simulink model "P3"  (Simulink 7.6)
settings: Solver=ode45  StartTime=0.0  StopTime=10.0  RelTol=1e-3
settings Model: Creator=USUARIO  LastModifiedBy=USUARIO

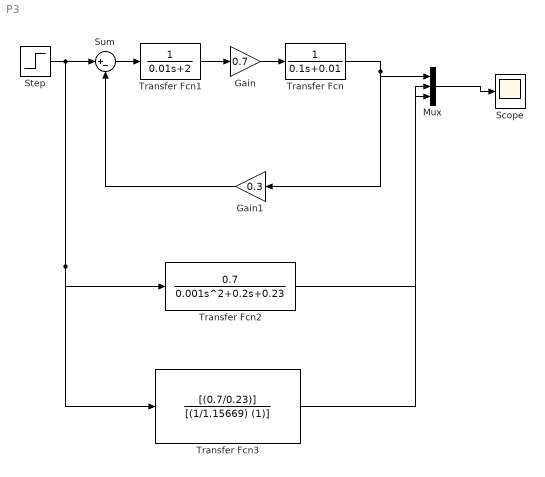
== system P3 ==
  Gain : Gain  Gain=0.7
  Gain1 : Gain  Gain=0.3
  Mux : Mux  Inputs=3
  Scope : Scope
  Step : Step  SampleTime=0
  Sum : Sum  Inputs=|+-
  Transfer Fcn : TransferFcn  Denominator=[0.1 0.01]
  Transfer Fcn1 : TransferFcn  Denominator=[0.01 2]
  Transfer Fcn2 : TransferFcn  Numerator=[0.7]  Denominator=[0.001 0.2 0.23]
  Transfer Fcn3 : TransferFcn  Numerator=[(0.7/0.23)]  Denominator=[(1/1.15669) (1)]
  wires:
  Step/1 -> Sum/1, Transfer Fcn2/1, Transfer Fcn3/1
  Sum/1 -> Transfer Fcn1/1
  Transfer Fcn1/1 -> Gain/1
  Gain/1 -> Transfer Fcn/1
  Transfer Fcn/1 -> Gain1/1, Mux/1
  Gain1/1 -> Sum/2
  Mux/1 -> Scope/1
  Transfer Fcn2/1 -> Mux/2
  Transfer Fcn3/1 -> Mux/3
